simulink subsystem "Automotive_PowerTrain"  (R2024a)
settings: Solver=VariableStepAuto  StartTime=0.0  StopTime=10.0  RelTol=1e-3
libraries: autolibsharedcoupling x4
settings Model: Creator=USER  LastModifiedBy=USER

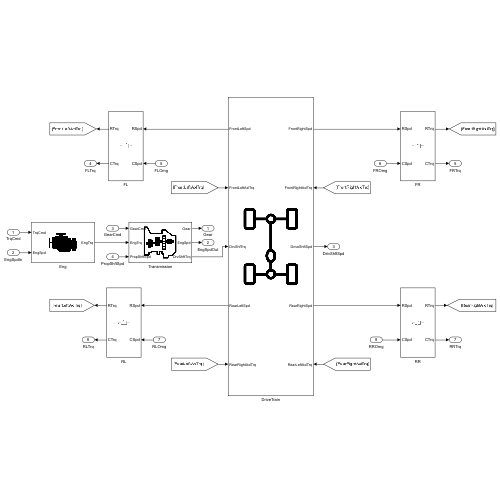
[thumbnail: Simulink's stored preview of the top-level diagram]
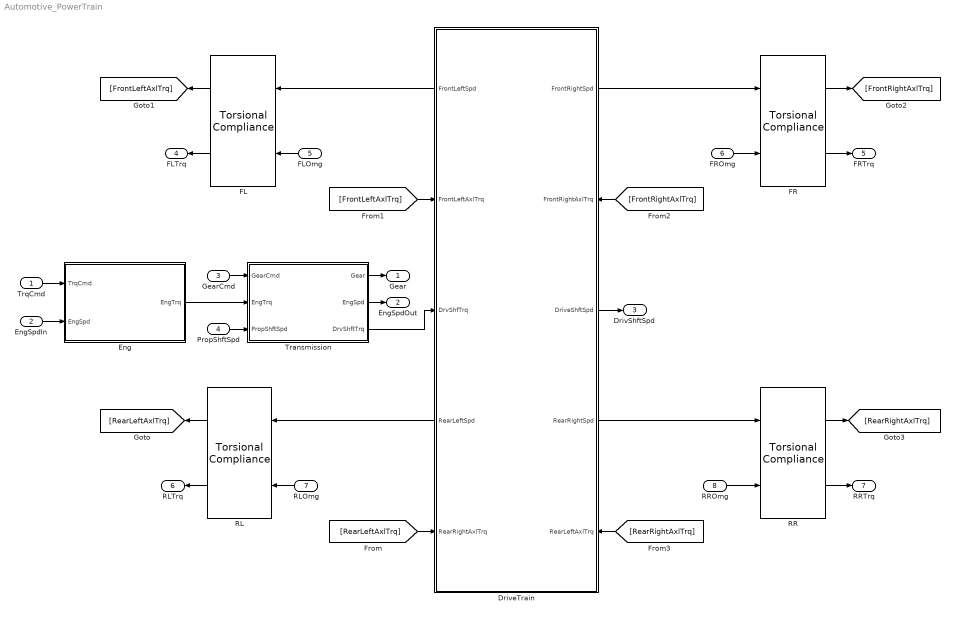
== system Automotive_PowerTrain ==
  TrqCmd : Inport
  EngSpdIn : Inport  Port=2
  GearCmd : Inport  Port=3
  PropShftSpd : Inport  Port=4
  FLOmg : Inport  Port=5
  FROmg : Inport  Port=6
  RLOmg : Inport  Port=7
  RROmg : Inport  Port=8
  DriveTrain : Subsystem
      settings: PortSchema="{\"entries\":[{\"content\":{\"sides\":[{\"content\":{\"connectorIds\":[\"Out4\",\"In1\",\"In2\",\"Out5\",\"In3\"]},\"type\":\"ConnectorPlacement.EquallySpacedRectSide\",\"uuid\":\"99dc967c-1fb5-417d-adc0-f46980eb8e16\"},{\"content\":{\"connectorIds\":[\"Out1\",\"In4\",\"Out2\",\"Out3\",\"In5\"],\"side\":\"RIGHT\"},\"type\":\"ConnectorPlacement.EquallySpacedRectSide\",\"uuid\":\"01a97c2b-f3cf-42df-9ac4-0ed5f444ed57\"},{\"content\":{\"side\":\"TOP\"},\"type\":\"ConnectorPlacement.EquallySpacedRectSide\",\"uuid\":\"79436a5a-4a01-4144-8a57-0ba821c66b11\"}]},\"type\":\"ConnectorPlacement.EquallySpacedConnector\",\"uuid\":\"41e95cf7-d1f1-497b-9f4f-e1586fb8f898\"}],\"packageUris\":[\"http://schema.mathworks.com/mf0/Connector/R2020b\"],\"version\":\"1.0\"}"
      mask Display: image('DriveTrainICon.png', [10,10,10,10,100,100]);
  Eng : Subsystem
      mask Display: image('EngIcon.png', [10,10,10,10,100,100]);
  FL : autolibsharedcoupling/Torsional Compliance  port_config=Simulink  extInfo=off  k=1e4  b=1e2  theta_o=0  domega_o=0  omega_c=3000  blkID=0  aMode=2
      settings: LibrarySourceBlock=vdynlib/Powertrain/Drivetrain/Couplings/Torsional Compliance
  FR : autolibsharedcoupling/Torsional Compliance  port_config=Simulink  extInfo=off  k=1e4  b=1e2  theta_o=0  domega_o=0  omega_c=3000  blkID=0  aMode=2
      settings: LibrarySourceBlock=vdynlib/Powertrain/Drivetrain/Couplings/Torsional Compliance
  RL : autolibsharedcoupling/Torsional Compliance  port_config=Simulink  extInfo=off  k=1e4  b=1e2  theta_o=0  domega_o=0  omega_c=3000  blkID=0  aMode=2
      settings: LibrarySourceBlock=vdynlib/Powertrain/Drivetrain/Couplings/Torsional Compliance
  RR : autolibsharedcoupling/Torsional Compliance  port_config=Simulink  extInfo=off  k=1e4  b=1e2  theta_o=0  domega_o=0  omega_c=3000  blkID=0  aMode=2
      settings: LibrarySourceBlock=vdynlib/Powertrain/Drivetrain/Couplings/Torsional Compliance
  Transmission : Subsystem
      mask Display: image('TransIcon.png', [10,10,10,10,100,100]);
  Gear : Outport
  EngSpdOut : Outport  Port=2
  DrivShftSpd : Outport  Port=3
  FLTrq : Outport  Port=4
  FRTrq : Outport  Port=5
  RLTrq : Outport  Port=6
  RRTrq : Outport  Port=7
  wires:
  DriveTrain/4(FrontLeftSpd) -> FL/1
  DriveTrain/1(FrontRightSpd) -> FR/1
  DriveTrain/5(RearLeftSpd) -> RL/1
  DriveTrain/3(RearRightSpd) -> RR/1
  Eng/1(EngTrq) -> Transmission/2(EngTrq)
  GearCmd/1 -> Transmission/1(GearCmd)
  PropShftSpd/1 -> Transmission/3(PropShftSpd)
  Transmission/1(Gear) -> Gear/1
  FL/2 -> FLTrq/1
  RL/2 -> RLTrq/1
  FR/2 -> FRTrq/1
  RR/2 -> RRTrq/1
  FLOmg/1 -> FL/2
  FROmg/1 -> FR/2
  RROmg/1 -> RR/2
  RLOmg/1 -> RL/2
  RL/1 -> [RearLeftAxlTrq]
  [RearLeftAxlTrq] -> DriveTrain/3(RearRightAxlTrq)
  FL/1 -> [FrontLeftAxlTrq]
  [FrontLeftAxlTrq] -> DriveTrain/1(FrontLeftAxlTrq)
  FR/1 -> [FrontRightAxlTrq]
  [FrontRightAxlTrq] -> DriveTrain/4(FrontRightAxlTrq)
  RR/1 -> [RearRightAxlTrq]
  [RearRightAxlTrq] -> DriveTrain/5(RearLeftAxlTrq)
  DriveTrain/2(DriveShftSpd) -> DrivShftSpd/1
  TrqCmd/1 -> Eng/1(TrqCmd)
  EngSpdIn/1 -> Eng/2(EngSpd)
  Transmission/2(EngSpd) -> EngSpdOut/1
  Transmission/3(DrvShftTrq) -> DriveTrain/2(DrvShfTrq)

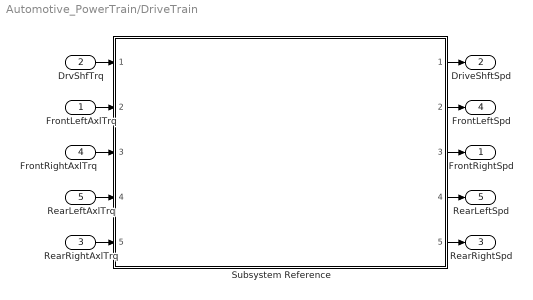
== system Automotive_PowerTrain/DriveTrain ==
  FrontLeftAxlTrq : Inport
  DrvShfTrq : Inport  Port=2
  RearRightAxlTrq : Inport  Port=3
  FrontRightAxlTrq : Inport  Port=4
  RearLeftAxlTrq : Inport  Port=5
  Subsystem Reference : Subsystem  ReferencedSubsystem=Automotive_PowerTrain_AWDDifferential
  FrontRightSpd : Outport
  DriveShftSpd : Outport  Port=2
  RearRightSpd : Outport  Port=3
  FrontLeftSpd : Outport  Port=4
  RearLeftSpd : Outport  Port=5
  wires:
  Subsystem Reference/5 -> RearRightSpd/1
  FrontRightAxlTrq/1 -> Subsystem Reference/3
  Subsystem Reference/3 -> FrontRightSpd/1
  Subsystem Reference/1 -> DriveShftSpd/1
  FrontLeftAxlTrq/1 -> Subsystem Reference/2
  DrvShfTrq/1 -> Subsystem Reference/1
  RearRightAxlTrq/1 -> Subsystem Reference/5
  RearLeftAxlTrq/1 -> Subsystem Reference/4
  Subsystem Reference/2 -> FrontLeftSpd/1
  Subsystem Reference/4 -> RearLeftSpd/1

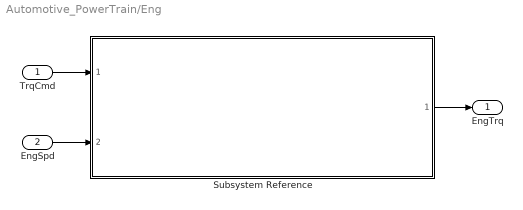
== system Automotive_PowerTrain/Eng ==
  TrqCmd : Inport
  EngSpd : Inport  Port=2
  Subsystem Reference : Subsystem  ReferencedSubsystem=Automotive_PowerTrain_SIEng
  EngTrq : Outport
  wires:
  TrqCmd/1 -> Subsystem Reference/1
  EngSpd/1 -> Subsystem Reference/2
  Subsystem Reference/1 -> EngTrq/1

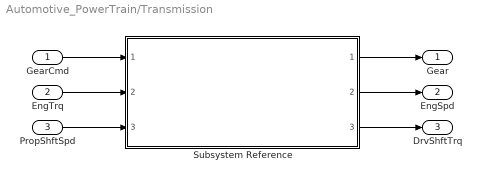
== system Automotive_PowerTrain/Transmission ==
  GearCmd : Inport
  EngTrq : Inport  Port=2
  PropShftSpd : Inport  Port=3
  Subsystem Reference : Subsystem  ReferencedSubsystem=Automotive_PowerTrain_Transmission
  Gear : Outport
  EngSpd : Outport  Port=2
  DrvShftTrq : Outport  Port=3
  wires:
  GearCmd/1 -> Subsystem Reference/1
  EngTrq/1 -> Subsystem Reference/2
  PropShftSpd/1 -> Subsystem Reference/3
  Subsystem Reference/1 -> Gear/1
  Subsystem Reference/2 -> EngSpd/1
  Subsystem Reference/3 -> DrvShftTrq/1
